simulink model "L2_2"  (Simulink 6.0)
settings: Solver=ode45  StartTime=0.0  StopTime=20.0  RelTol=1e-3
undefined symbols (not defined in the file): k, Ti
settings Model: LastModifiedBy=student

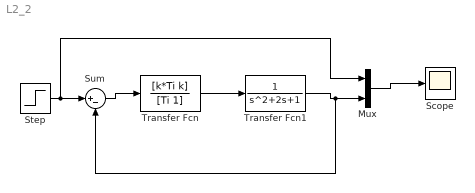
== system L2_2 ==
  Mux : Mux  Inputs=2
  Scope : Scope
      settings: TimeRange=10  YMin=0.906968  YMax=0.909456
  Step : Step  SampleTime=0
  Sum : Sum  Inputs=|+-
  Transfer Fcn : TransferFcn  Numerator=[k*Ti k]  Denominator=[Ti 1]
  Transfer Fcn1 : TransferFcn
  wires:
  Step/1 -> Sum/1, Mux/1
  Mux/1 -> Scope/1
  Transfer Fcn1/1 -> Mux/2, Sum/2
  Transfer Fcn/1 -> Transfer Fcn1/1
  Sum/1 -> Transfer Fcn/1
